simulink model "Model_nie_liniowy_zapiete_sprzerzenie"  (R2017a)
settings: Solver=ode45  StartTime=0.0  StopTime=50  FixedStep=0.01  MaxStep=0.0001  RelTol=1e-3  EnableMultiTasking=on
values from neighbouring files (symbols this model uses):
  L1 = L_calka(1:2, 1:4)    [Linearyzacja_ramienia_robota.m]
  L2 = L_calka(1:2, 5:6)    [Linearyzacja_ramienia_robota.m]
  M = inv(C * (B * L - A)^-1 * B)    [Linearyzacja_ramienia_robota.m]
libraries: commchan3 x4
settings Model: Creator=kss  LastModifiedBy=Pankiev
settings SolverCC: MaxConsecutiveZCs=100000  ZeroCrossControl=EnableAll  SolverResetMethod=Robust
settings OptimizationCC: LifeSpan=inf
settings DebuggingCC: SFUnexpectedBacktrackingDiag=warning  SFNoUnconditionalDefaultTransitionDiag=warning  SFExecutionAtInitializationDiag=none
settings GRTTargetCC: TargetLangStandard=C89/C90 (ANSI)  GeneratePreprocessorConditionals=Disable all
settings ConfigComp: CovMetricSettings=dw  CovHtmlReporting=on  CovSaveCumulativeToWorkspaceVar=on  CovSaveSingleToWorkspaceVar=on  CovExternalEMLEnable=off

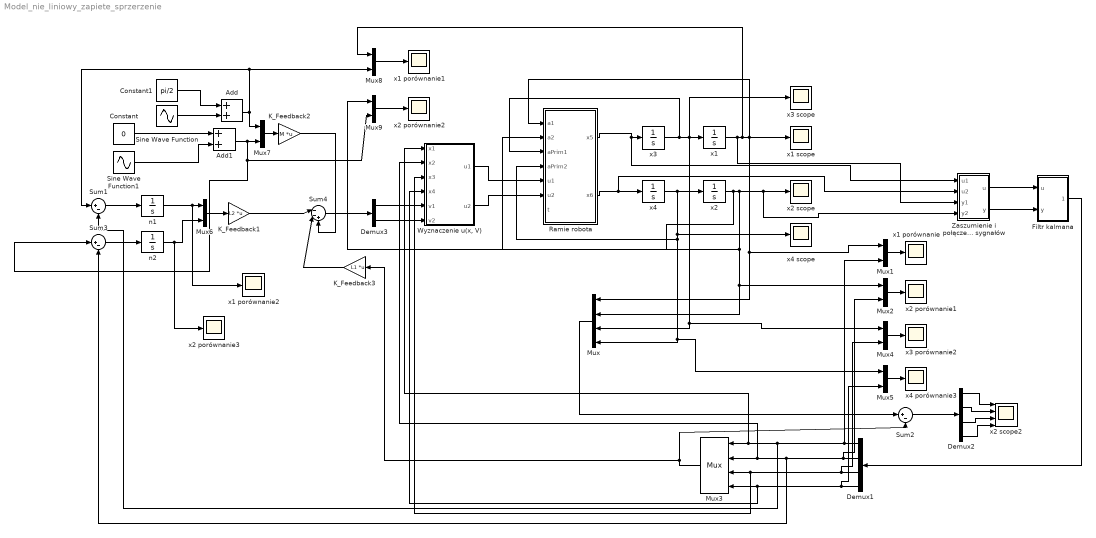
== system Model_nie_liniowy_zapiete_sprzerzenie ==
  Add : Sum
  Add1 : Sum
  Constant : Constant  Value=0
  Constant1 : Constant  Value=pi/2
  Demux1 : Demux
  Demux2 : Demux
  Demux3 : Demux  Outputs=2
  Filtr kalmana : Subsystem
  K_Feedback1 : Gain  Gain=L2  Multiplication=Matrix(K*u)
  K_Feedback2 : Gain  Gain=M  Multiplication=Matrix(K*u)
  K_Feedback3 : Gain  Gain=L1  Multiplication=Matrix(K*u)
  Mux : Mux
  Mux{1..2,4..9} (8 alike) : Mux  Inputs=2
  Mux3 : Mux
      settings: DisplayOption=signals
  Ramie robota : MATLAB Function  TreatAsAtomicUnit=on
  Sine Wave Function : Sin  SampleTime=0
  Sine Wave Function1 : Sin  Phase=pi/2  SampleTime=0
  Sum1 : Sum  Inputs=|+-
  Sum2 : Sum  Inputs=|+-
  Sum3 : Sum  Inputs=|+-
  Sum4 : Sum  Inputs=|--+
  "Wyznaczenie u(x, V)" : MATLAB Function  TreatAsAtomicUnit=on
  Zaszumienie i połączenie sygnałów : Subsystem
  n1 : Integrator  InitialCondition=0.3  AbsoluteTolerance=1e-5
  n2 : Integrator  InitialCondition=0.3  AbsoluteTolerance=1e-5
  x1 : Integrator  InitialCondition=(pi/2)-0.3  AbsoluteTolerance=1e-5
  x1 porównanie : Scope
  x1 porównanie1 : Scope
  x1 porównanie2 : Scope
  x1 scope : Scope
  x2 : Integrator  InitialCondition=0.3  AbsoluteTolerance=1e-5
  x2 porównanie1 : Scope
  x2 porównanie2 : Scope
  x2 porównanie3 : Scope
  x2 scope : Scope
  x2 scope2 : Scope  NumInputPorts=4
  x3 : Integrator  AbsoluteTolerance=1e-5
  x3 porównanie2 : Scope
  x3 scope : Scope
  x4 : Integrator  AbsoluteTolerance=1e-5
  x4 porównanie3 : Scope
  x4 scope : Scope
  wires:
  Ramie robota/1(x5) -> Zaszumienie i połączenie sygnałów/1(u1), x3/1
  Ramie robota/2(x6) -> Zaszumienie i połączenie sygnałów/2(u2), x4/1
  x3/1 -> Ramie robota/3(aPrim1), x3 scope/1, Mux4/1, Mux/3, x1/1
  x4/1 -> x4 scope/1, Mux5/1, Mux/4, Ramie robota/4(aPrim2), x2/1
  x1/1 -> Zaszumienie i połączenie sygnałów/3(y1), Mux8/1, Mux/1, Mux1/1, x1 scope/1, Ramie robota/1(a1)
  Demux1/1 -> Sum1/2, "Wyznaczenie u(x, V)"/1(x1), Mux3/1, Mux1/2
  Demux1/2 -> Mux2/2, Sum3/2, "Wyznaczenie u(x, V)"/2(x2), Mux3/2
  Demux1/3 -> Mux4/2, "Wyznaczenie u(x, V)"/3(x3), Mux3/3
  Filtr kalmana/1(Out1) -> Demux1/1
  Zaszumienie i połączenie sygnałów/1(u) -> Filtr kalmana/1(u)
  Zaszumienie i połączenie sygnałów/2(y) -> Filtr kalmana/2(y)
  Mux1/1 -> x1 porównanie/1
  Mux3/1 -> K_Feedback3/1, Sum2/2
  Mux/1 -> Sum2/1
  Mux2/1 -> x2 porównanie1/1
  Mux4/1 -> x3 porównanie2/1
  Mux5/1 -> x4 porównanie3/1
  Sum2/1 -> Demux2/1
  Demux2/2 -> x2 scope2/2
  Demux2/3 -> x2 scope2/3
  Demux2/4 -> x2 scope2/4
  Demux2/1 -> x2 scope2/1
  Mux6/1 -> K_Feedback1/1
  n2/1 -> x2 porównanie3/1, Mux6/2
  n1/1 -> x1 porównanie2/1, Mux6/1
  x2/1 -> Mux9/1, Zaszumienie i połączenie sygnałów/4(y2), x2 scope/1, Mux2/1, Mux/2, Ramie robota/2(a2)
  Demux3/1 -> "Wyznaczenie u(x, V)"/5(v1)
  Demux3/2 -> "Wyznaczenie u(x, V)"/6(v2)
  "Wyznaczenie u(x, V)"/2(u2) -> Ramie robota/6(u2)
  "Wyznaczenie u(x, V)"/1(u1) -> Ramie robota/5(u1)
  Demux1/4 -> Mux5/2, "Wyznaczenie u(x, V)"/4(x4), Mux3/4
  K_Feedback3/1 -> Sum4/2
  Sum4/1 -> Demux3/1
  Mux7/1 -> K_Feedback2/1
  Constant1/1 -> Add/1
  Add1/1 -> Mux9/2, Sum3/1, Mux7/2
  Add/1 -> Mux7/1, Mux8/2, Sum1/1
  Constant/1 -> Add1/1
  Sum1/1 -> n1/1
  Sum3/1 -> n2/1
  K_Feedback1/1 -> Sum4/1
  Sine Wave Function/1 -> Add/2
  Sine Wave Function1/1 -> Add1/2
  K_Feedback2/1 -> Sum4/3
  Mux8/1 -> x1 porównanie1/1
  Mux9/1 -> x2 porównanie2/1

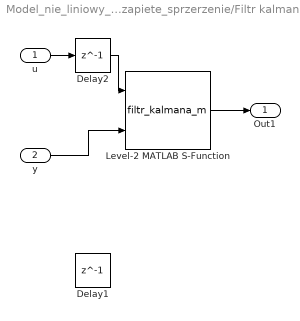
== system Model_nie_liniowy_zapiete_sprzerzenie/Filtr kalmana ==
  u : Inport
  y : Inport  Port=2
  Delay1 : Delay  DelayLength=1  InitialCondition=[pi/2-0.3;0.3]  SampleTime=0.0001
  Delay2 : Delay  DelayLength=1  SampleTime=0.0001
  Level-2 MATLAB S-Function : M-S-Function  FunctionName=filtr_kalmana_m  Parameters=[(pi/2)-0.3; 0.3; 0; 0]
  Out1 : Outport
  wires:
  Level-2 MATLAB S-Function/1 -> Out1/1
  u/1 -> Delay2/1
  Delay2/1 -> Level-2 MATLAB S-Function/1
  y/1 -> Level-2 MATLAB S-Function/2

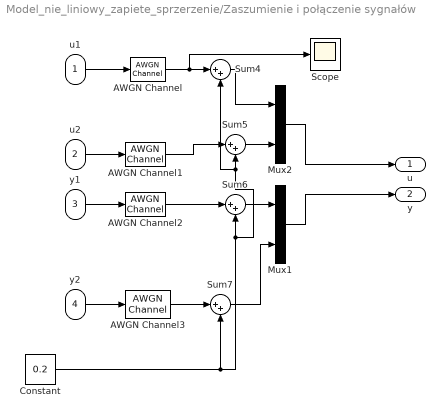
== system Model_nie_liniowy_zapiete_sprzerzenie/Zaszumienie i połączenie sygnałów ==
  u1 : Inport  SampleTime=0.001
  u2 : Inport  Port=2  SampleTime=0.001
  y1 : Inport  Port=3  SampleTime=0.001
  y2 : Inport  Port=4  SampleTime=0.001
  AWGN Channel : commchan3/AWGN Channel  InputProcessing=Columns as channels (frame based)  seed=1234  noiseMode="Signal to noise ratio  (Es/No)"  EbNodB=10  EsNodB=-10  SNRdB=10  bitsPerSym=1  Ps=10^-4  Tsym=0.01  variance=1
  AWGN Channel1 : commchan3/AWGN Channel  InputProcessing=Columns as channels (frame based)  seed=53467  noiseMode="Signal to noise ratio  (Es/No)"  EbNodB=10  EsNodB=-10  SNRdB=10  bitsPerSym=1  Ps=10^-4  Tsym=0.01  variance=1
  AWGN Channel2 : commchan3/AWGN Channel  InputProcessing=Columns as channels (frame based)  seed=57621  noiseMode="Signal to noise ratio  (Es/No)"  EbNodB=10  EsNodB=-10  SNRdB=10  bitsPerSym=1  Ps=10^-4  Tsym=0.01  variance=1
  AWGN Channel3 : commchan3/AWGN Channel  InputProcessing=Columns as channels (frame based)  seed=92523  noiseMode="Signal to noise ratio  (Es/No)"  EbNodB=10  EsNodB=-10  SNRdB=10  bitsPerSym=1  Ps=10^-4  Tsym=0.01  variance=1
  Constant : Constant  Value=0.2
  Mux1 : Mux  Inputs=2
  Mux2 : Mux  Inputs=2
  Scope : Scope
  Sum{4..7} (4 alike) : Sum  Inputs=|++
  u : Outport
  y : Outport  Port=2
  wires:
  Sum5/1 -> Mux2/2
  Sum7/1 -> Mux1/2
  Mux2/1 -> u/1
  Mux1/1 -> y/1
  Sum4/1 -> Mux2/1
  Sum6/1 -> Mux1/1
  Constant/1 -> Sum7/2, Sum4/2, Sum5/2, Sum6/2
  y2/1 -> AWGN Channel3/1
  AWGN Channel3/1 -> Sum7/1
  y1/1 -> AWGN Channel2/1
  AWGN Channel2/1 -> Sum6/1
  u2/1 -> AWGN Channel1/1
  AWGN Channel1/1 -> Sum5/1
  u1/1 -> AWGN Channel/1
  AWGN Channel/1 -> Scope/1, Sum4/1

== matlab function Model_nie_liniowy_zapiete_sprzerzenie/Wyznaczenie u(x, V) ==
  data: x1 input; u1 output; x2 input; x3 input; x4 input; v1 input; v2 input; u2 output
function [u1, u2] = fcn(x1, x2, x3, x4, v1, v2)

m1 = 2;
m2 = 1;
L1 = 1.5;
L2 = 1;
Lc1 = L1/2;
Lc2 = L2/2;
J1 = (m1*L1^2)/3;
J2 = (m2*L2^2)/3;
g = 9.81;

H11 = m1 * Lc1^2 + J1 + m2 * (L1^2 + Lc2^2 + 2 * L1 * L2 * cos(x2)) + J2;
H12  = m2 * L1 * Lc2 * cos(x2) + m2 * Lc2^2 + J2;
H21 = H12;
H22 = m2 * Lc2^2 + J2;

h = m2 * L1 * Lc2 * sin(x2);
g1 = m1 * Lc1 * g * cos(x1) + m2 * g * (Lc2 * cos(x1+x2) + L1 * cos(x1));
g2 = m2 * Lc2 * g * cos(x1+x2);

H = [H11 H12;
     H21 H22];

J = [-h * x4, -h * x3 - h *x4;
     h*x3, 0];
M = [g1;
     g2];
V = [v1;
     v2];
F = J * [x3; x4] + M;

T = H * V + F;
u1 = T(1);
u2 = T(2);

== matlab function Model_nie_liniowy_zapiete_sprzerzenie/Ramie robota ==
  data: a1 input; a2 input; aPrim1 input; aPrim2 input; u1 input; u2 input; x5 output; x6 output; t input
function [x5,x6] = fcn(a1,a2,aPrim1,aPrim2,u1,u2,t)
m1 = 2; m2 = 1 * 1.15; l1 = 1.5; l2 = 1; lc1 = l1/2; lc2 = l2/2; J1 = (m1*l1^2)/3; J2 = (m2*l2^2)/3; g = 9.81;
H11 = m1*lc1^2 + J1 + m2*(l1^2 + lc2^2 + 2*l1*l2*cos(a2)) + J2;
H12  = m2*l1*lc2*cos(a2) + m2*lc2^2 + J2;
H21 = H12;
H22 = m2*lc2^2 + J2;
h = m2*l1*lc2*sin(a2);
g1 = m1*lc1*g*cos(a1) + m2*g*(lc2*cos(a1+a2)+l1*cos(a1));
g2 = m2*lc2*g*cos(a1+a2);
H = [H11 H12; H21 H22];
H2 = inv(H);
Z = [0;0];

J = [-h*aPrim2, -h*aPrim1-h*aPrim2; h*aPrim1,0];
M = [g1;g2];
U = [u1;u2];
%rozwikłanie 
Roz = -1*H2*J*[aPrim1; aPrim2] -1*H2*M + H2*U + H2 * Z; 
x5 = Roz(1);
x6 = Roz(2);
% x5 = (200*T1 - 200*T2 + (2943*cos(x1 + 2*x2))/2 - (8829*cos(x1))/2 + 150*x3^2*sin(x2) + 150*x4^2*sin(x2) + 225*x3^2*sin(2*x2) - 23544*J2*cos(x1) - 600*T2*cos(x2) + 800*J2*T1 - 800*J2*T2 + 300*x3*x4*sin(x2) + 600*J2*x3^2*sin(x2) + 600*J2*x4^2*sin(x2) + 1200*J2*x3*x4*sin(x2))/(25*(8*J1 + 108*J2 - 9*cos(2*x2) + 32*J1*J2 + 18));
% x6 = -(400*T1 - 5800*T2 - 17658*cos(x1 - x2) + 2943*cos(x1 + 2*x2) + 8829*cos(x1 + x2) - 8829*cos(x1) + 4350*x3^2*sin(x2) + 300*x4^2*sin(x2) + 7848*J1*cos(x1 + x2) + 900*x3^2*sin(2*x2) + 450*x4^2*sin(2*x2) - 47088*J2*cos(x1) + 1200*T1*cos(x2) - 2400*T2*cos(x2) - 1600*J1*T2 + 1600*J2*T1 - 1600*J2*T2 + 600*x3*x4*sin(x2) + 1200*J1*x3^2*sin(x2) + 1200*J2*x3^2*sin(x2) + 1200*J2*x4^2*sin(x2) + 900*x3*x4*sin(2*x2) + 2400*J2*x3*x4*sin(x2))/(50*(8*J1 + 108*J2 - 9*cos(2*x2) + 32*J1*J2 + 18));

%y = u;
